simulink model "CaptureOutputs_roe"  (R2018b)
settings: Solver=ode4  StartTime=0.0  StopTime=SimEndTime  FixedStep=TimeStep  RelTol=1e-3
model workspace (MATLAB code in the model file):
  | CON = Simulink.Parameter;
  | CON.DataType = 'Bus: Bus_CON';
  | CON.Value = Simulink.Bus.createMATLABStruct('Bus_CON');
undefined symbols (not defined in the file): SampleTime, TimeStep
settings Model: ParameterArgumentNames=CON  OrderedModelArguments=off  Creator=Ethan  LastModifiedBy=Ethan
settings ModelReferenceCC: ModelReferenceNumInstancesAllowed=Single

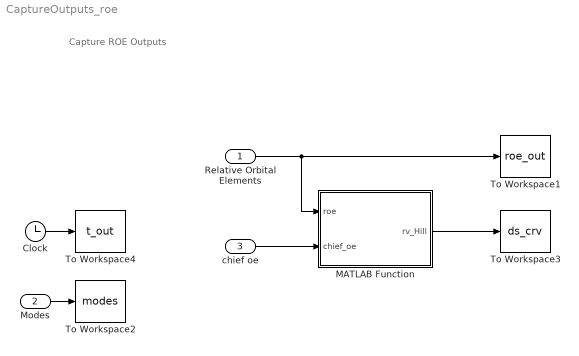
== system CaptureOutputs_roe ==
  note: Capture ROE Outputs
  Relative Orbital Elements : Inport  PortDimensions=7  SampleTime=TimeStep
  Modes : Inport  Port=2  OutDataTypeStr=Bus: Bus_modes  PortDimensions=1  SampleTime=TimeStep  BusOutputAsStruct=on
  chief oe : Inport  Port=3  OutDataTypeStr=Bus: Bus_OE
  Clock : Clock
  MATLAB Function : MATLAB Function  TreatAsAtomicUnit=on
  To Workspace1 : ToWorkspace  VariableName=roe_out  SampleTime=SampleTime
      settings: Save2DSignal=2-D array (concatenate along first dimension)
  To Workspace2 : ToWorkspace  VariableName=modes  SaveFormat=Timeseries  SampleTime=SampleTime
      settings: Save2DSignal=2-D array (concatenate along first dimension)
  To Workspace3 : ToWorkspace  VariableName=ds_crv  SampleTime=SampleTime
      settings: Save2DSignal=2-D array (concatenate along first dimension)
  To Workspace4 : ToWorkspace  VariableName=t_out  SampleTime=SampleTime
      settings: Save2DSignal=2-D array (concatenate along first dimension)
  wires:
  Relative Orbital Elements/1 -> MATLAB Function/1(roe), To Workspace1/1
  Clock/1 -> To Workspace4/1
  Modes/1 -> To Workspace2/1
  chief oe/1 -> MATLAB Function/2(chief_oe)
  MATLAB Function/1(rv_Hill) -> To Workspace3/1

== matlab function CaptureOutputs_roe/MATLAB Function ==
  data: roe input; chief_oe input; rv_Hill output
function rv_Hill = roe2Hill(roe, chief_oe)

da = roe(2);
dL = roe(3);
dex = roe(4);
dey = roe(5);
dix = roe(6);
diy = roe(7);

ad = da * chief_oe.a + chief_oe.a;
edx = dex + chief_oe.e * cosd(chief_oe.w);
edy = dey + chief_oe.e * sind(chief_oe.w);

ed = sqrt(edx ^ 2 + edy ^ 2);

id = dix * 180 / pi + chief_oe.inc;

od = diy / sind(chief_oe.inc) * 180 / pi + chief_oe.omega;
wd = atan2d(edy, edx);
% wd = 0;
ud = dL * 180/pi - diy*180/pi/sind(chief_oe.inc) * cosd(chief_oe.inc) + (chief_oe.nu + chief_oe.w);
nud = ud - wd;
[rTgt,vTgt] = oe2rvECI(chief_oe.a, chief_oe.e, chief_oe.inc, chief_oe.omega,...
    chief_oe.w, chief_oe.nu);
[rChase,vChase] = oe2rvECI(ad,ed,id,od,wd,nud);

[rHill,vHill] = ECI2Hill_Vectorized(rTgt,vTgt,rChase,vChase);

rv_Hill = [rHill; vHill];
